simulink model "testdelay"  (Simulink 7.5)
settings: Solver=ode1  StartTime=0.0  StopTime=6  FixedStep=T  RelTol=1e-3
PreLoadFcn:
  | T=0.005;
settings Model: Creator=gcampa  LastModifiedBy=it
settings DataIOCC: LimitDataPoints=off  SaveOutput=off  SignalLogging=off
settings DebuggingCC: SaveWithParameterizedLinksMsg=none  MultiTaskCondExecSysMsg=none  StrictBusMsg=Warning
settings HardwareCC: TargetHWDeviceType=32-bit Generic
settings RTWCC: IncludeERTFirstTime=on
settings GRTTargetCC: TargetFcnLib=ansi_tfl_tmw.mat

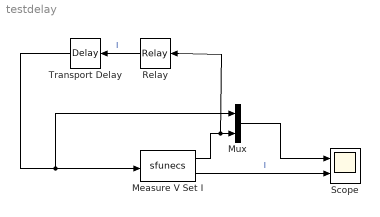
== system testdelay ==
  Measure V Set I : S-Function  FunctionName=sfunecs  Parameters=idx,m,ab,T  EnableBusSupport=off  mask(ECS Board Block){idx=0, m=off, ab=[1 0 ], T=-1}
      mask prompts: idx "Board Index [0,19]"; m "Set Current"; ab "Current Scaling [a b] (i=a*vx+b)"; T "Sampling Time (-1 = Inherited)"
      mask help:
      | This block controls the Olin ECS Board.
      | At each sample time, the block takes the scalar value at its input and uses it to set the output voltage across the terminals of the indexed board. If the Set Current checkbox is checked, the input value is interpreted as a current and used to set the current flowing trough the terminals.
      | The first output is the measured voltage across the terminals in volts, the second one is the measured current flowing trough the terminals. Note that the current is set by regulating an internal voltage vx (in volts) which is mapped to the current according to the scaling parameters a and b (i=a*vx+b). Set a=1 and b=0 to have i=vx, so that vx can be regulated and measured directly.
      mask Help:
      | <p>
      | This block controls the Olin ECS Board.
      | </p>
      | <p>
      | At each sample time, the block takes the scalar value at its input and uses it to set the output voltage across the terminals of the indexed board. If the Set Current checkbox is checked, the input value is interpreted as a current and used to set the current flowing trough the terminals.
      | The first output is the measured voltage across the terminals in volts, the second one is the measured current flowing trough the terminals. Note that the current is set by regulating an internal voltage vx (in volts) which is mapped to the current according to the scaling parameters a and b (i=a*vx+b).Set a=1 and b=0 to have i=vx, so that vx can be regulated and measured directly.
      | </p>
  Mux : Mux  Inputs=2
  Relay : Relay  OnOutputValue=-1  OffOutputValue=1  OutDataType=fixdt(1, 16)  OutScaling=2^0
  Scope : Scope  NumInputPorts=2
      settings: YMin=-12.5~-0.012  YMax=12.5~0.009
  Transport Delay : TransportDelay  DelayTime=0.1
  wires:
  Relay/1 -> Transport Delay/1  "I"
  Measure V Set I/2 -> Scope/2  "I"
  Measure V Set I/1 -> Mux/2, Relay/1
  Mux/1 -> Scope/1
  Transport Delay/1 -> Measure V Set I/1, Mux/1
